simulink model "NavigationRocketPlant"  (R2025b)
settings: Solver=ode5  StartTime=0.0  StopTime=350  RelTol=1e-3
PostLoadFcn:
  | addpath('settings/')
  | addpath('settings/environment/')
  | 
  | run sensorSettings.m
InitFcn:
  | run(fullfile(fileparts(get_param(bdroot,'FileName')),'..','rocketPlantMain.m'))
values from neighbouring files (symbols this model uses):
  Rocket = block.DialogPrm(1).Data    [rocketPlantBlock.m]
  Weather = block.DialogPrm(3).Data    [rocketPlantBlock.m]
undefined symbols (not defined in the file or in its folder): ba0, bg0, DiscIntNeverNeededParam, dspblkCoreblockFVToolHelper, Environment, gcbh, GNSSConfig, GNSSInitialState, LLA0, MEKF, p0, P0, pressure0, q0, RocketInitialState, Sensor, stationaryTime, v0
libraries: simulink x2, dspmathops x1
(part 3 of 3)

== matlab function NavigationRocketPlant/Navigation/State Estimation/MEKF ==
  settings: updateMethod=DISCRETE  sampleTime=Sensor.Ts
  data: dt input; q_nb_out output; gyro_b input; acc_b input; baro_pressure_Pa input; mag_b input; h0_m input; gps_pos_n input; gps_fix_info input; mag_ref_n input; q_nb_in input; v_n_in input; p_n_in input; bg_in input; ba_in input; P_in input; use_acc_tilt input; mag_valid input; baro_valid input; gps_valid input; gps_frequency_Hz input; gps_timer_in input; v_n_out output; p_n_out output; bg_out output; ba_out output; P_out output; estimate_bias input; zeroUpdate input; gps_timer_out output; MEKF parameter; gps_diagnostic_out output; baro_calibration_out output double size=[2 1]; baro_calibration_in input double size=[2 1]; GNSSConfig parameter
function [q_nb_out, v_n_out, p_n_out, bg_out, ba_out, P_out, gps_timer_out, gps_diagnostic_out, baro_calibration_out] = MEKF_Navigation( ...
    dt, gyro_b, acc_b, baro_pressure_Pa, mag_b, h0_m, ...
    gps_pos_n, gps_fix_info, mag_ref_n, ...
    q_nb_in, v_n_in, p_n_in, bg_in, ba_in, P_in, ...
    use_acc_tilt, mag_valid, baro_valid, gps_valid, ...
    gps_frequency_Hz, gps_timer_in, ...
    estimate_bias, zeroUpdate, MEKF, baro_calibration_in, GNSSConfig)

    % -------------------------------------------------------------------------
    % Multiplicative Extended Kalman Filter for Navigation
    %
    % Sensors:
    %   gyro_b            : 3-axis gyroscope [rad/s]
    %   acc_b             : 3-axis accelerometer [m/s^2]
    %   mag_b             : 3-axis magnetometer [arbitrary unit or tesla]
    %   baro_pressure_Pa  : barometer pressure [Pa]
    %   gps_pos_n         : optional GPS position in local NED [m]
    %   gps_fix_info      : fresh/valid/acquisition time/age/NED sigma/status
    %   gps_frequency_Hz  : GPS update frequency [Hz]
    %   gps_timer_in      : last processed acquisition timestamp [s]
    %
    % Frame:
    %   n : local NED navigation frame
    %   b : body frame
    %
    % Quaternion:
    %   q_nb = [qx; qy; qz; qw], scalar-last
    %   q_nb maps body-frame vectors into navigation-frame vectors
    %
    % Nominal state:
    %   q_nb : attitude quaternion
    %   v_n  : velocity in NED [m/s]
    %   p_n  : position in NED [m]
    %   bg   : gyro bias [rad/s]
    %   ba   : accelerometer bias [m/s^2]
    %
    % Error state:
    %   dx = [dtheta; dv; dp; dbg; dba] in R^15
    %
    % Local NED convention:
    %   p_n(3) = D
    %   source-datum absolute altitude = h0_m - D
    %
    % -------------------------------------------------------------------------
    
    % -------------------------------------------------------------------------
    % Constants
    % -------------------------------------------------------------------------
    
    g0 = 9.80665;        % gravity magnitude [m/s^2]
    
    % -------------------------------------------------------------------------
    % Process diffusion tuning: Qd = G*Qc*G'*dt
    % -------------------------------------------------------------------------
    
    sigma_g = MEKF.sigma_g;
    sigma_a = MEKF.sigma_a;
    sigma_bg = MEKF.sigma_bg;
    sigma_ba = MEKF.sigma_ba;
    
    % -------------------------------------------------------------------------
    % Measurement-noise tuning
    % -------------------------------------------------------------------------
    
    sigma_acc_tilt = MEKF.sigma_acc_tilt;
    sigma_mag = MEKF.sigma_mag;
    sigma_baro_p = MEKF.sigma_baro_p;
    
    % Accelerometer update gate.
    % Accelerometer is used as gravity direction only when norm is close to g.
    acc_gate = MEKF.acc_gate;
    
    % -------------------------------------------------------------------------
    % Input protection
    % -------------------------------------------------------------------------
    
    if dt <= 0.0
        dt = 1.0e-3;
    end

    % -------------------------------------------------------------------------
    % GNSS delivery and duplicate/stale protection
    % -------------------------------------------------------------------------
    % A held receiver position is not a fresh measurement. Use the delivered
    % packet flags and timestamp, rather than a second independent 10 Hz timer.
    % Initialize the last processed timestamp to -1 so epoch zero is accepted.
    gps_timer = gps_timer_in;
    gps_update = 0;
    gps_age = gps_fix_info(4);
    gps_diagnostic = [0.0; 0.0; 0.0; gps_age];
    if gps_valid && gps_frequency_Hz > 0.0 && ...
            gps_fix_info(1) > 0.5 && gps_fix_info(2) > 0.5 && ...
            all(isfinite(gps_fix_info)) && gps_age >= 0.0 && ...
            gps_age <= GNSSConfig.MaxAge && ...
            gps_fix_info(3) > gps_timer_in + 1.0e-9 && ...
            all(gps_fix_info(5:7) >= 0.0)
        gps_update = 1;
        gps_timer = gps_fix_info(3);
        gps_diagnostic(1) = 1.0;
    end
    
    q_nb = quatNormalize(q_nb_in);
    v_n  = v_n_in;
    p_n  = p_n_in;
    bg   = bg_in;
    ba   = ba_in;
    

    P = 0.5 * (P_in + P_in');
    % Startup pressure zeroing at the known local origin.
    % Explicit Unit Delay state [offset_Pa; sample_count], initially [0;0].
    % Reset each simulation; freeze at launch. No sensor truth is used.
    baro_offset_Pa = baro_calibration_in(1);
    baro_samples = baro_calibration_in(2);
    if MEKF.baro_zero_enabled && zeroUpdate && baro_valid && isfinite(baro_pressure_Pa)
        [p_origin, ~] = ISA_model(0.0, h0_m);
        baro_samples = baro_samples + 1.0;
        baro_offset_Pa = baro_offset_Pa + ...
            (baro_pressure_Pa - p_origin - baro_offset_Pa) / baro_samples;
    end
    baro_pressure_calibrated = baro_pressure_Pa;
    if MEKF.baro_zero_enabled
        baro_pressure_calibrated = baro_pressure_Pa - baro_offset_Pa;
    end
    baro_calibration_out = [baro_offset_Pa; baro_samples];

    
    % -------------------------------------------------------------------------
    % Prediction step
    % -------------------------------------------------------------------------
    
    omega_b = gyro_b - bg;
    f_b     = acc_b  - ba;
    
    % Quaternion propagation.
    dq = deltaQuat(omega_b * dt);
    q_nb = quatNormalize(quatMultiply(q_nb, dq));
    
    % Rotation matrix from body frame to navigation frame.
    C_nb = quatToDcm(q_nb);
    
    % Strapdown translational propagation.
    % In NED, gravity is positive in the Down direction.
    g_n = [0.0; 0.0; g0];
    
    a_n = C_nb * f_b + g_n;
    
    p_n = p_n + v_n * dt + 0.5 * a_n * dt * dt;
    v_n = v_n + a_n * dt;
    
    % -------------------------------------------------------------------------
    % Covariance prediction
    % -------------------------------------------------------------------------
    
    F = zeros(15,15);
    
    % Attitude error dynamics:
    % dtheta_dot = -skew(omega_b) dtheta - dbg
    F(1:3,1:3)   = -skew3(omega_b);
    F(1:3,10:12) = -eye(3);
    
    % Velocity error dynamics:
    % dv_dot = -C_nb skew(f_b) dtheta - C_nb dba
    F(4:6,1:3)   = -C_nb * skew3(f_b);
    F(4:6,13:15) = -C_nb;
    
    % Position error dynamics:
    % dp_dot = dv
    F(7:9,4:6) = eye(3);
    
    % Bias dynamics:
    %   bg_dot = n_bg
    %   ba_dot = n_ba
    
    Phi = eye(15) + F * dt;
    
    G = zeros(15,12);
    
    G(1:3,1:3)     = -eye(3);   % gyro noise
    G(4:6,4:6)     = -C_nb;     % accelerometer noise
    G(10:12,7:9)   = eye(3);    % gyro bias random walk
    G(13:15,10:12) = eye(3);    % accelerometer bias random walk
    
    Qc = zeros(12,12);
    
    Qc(1:3,1:3)     = sigma_g^2  * eye(3);
    Qc(4:6,4:6)     = sigma_a^2  * eye(3);
    Qc(7:9,7:9)     = sigma_bg^2 * eye(3);
    Qc(10:12,10:12) = sigma_ba^2 * eye(3);
    
    Qd = G * Qc * G' * dt;
    
    P = Phi * P * Phi' + Qd;
    P = 0.5 * (P + P');

    
    if zeroUpdate
    
        [q_nb, v_n, p_n, bg, ba, P] = ZeroUpdateKalmanFilter( ...
            gyro_b, acc_b, q_nb, v_n, p_n, bg, ba, P, g0, estimate_bias, MEKF);
    
        C_nb = quatToDcm(q_nb);
    
    end

    % -------------------------------------------------------------------------
    % Accelerometer attitude update
    % -------------------------------------------------------------------------
    % The accelerometer update is used only when the acceleration norm is close
    % to gravity. Otherwise, the accelerometer contains significant translational
    % acceleration and should not be treated as a gravity vector.
    
    % Use the corrected bias; do not reuse the pre-zero-update value.
    f_b = acc_b - ba;
    acc_norm = norm3(f_b);
    
    if use_acc_tilt && ~zeroUpdate && acc_norm > 1.0e-6
    
        if abs(acc_norm - g0) < acc_gate * g0
    
            y_acc = f_b / acc_norm;
    
            C_bn = C_nb';
    
            g_unit_n = [0.0; 0.0; 1.0];
    
            % At rest, accelerometer measures approximately -gravity direction.
            yhat_acc = -C_bn * g_unit_n;
    
            H_acc = zeros(3,15);
            H_acc(:,1:3) = skew3(yhat_acc);
    
            [q_nb, v_n, p_n, bg, ba, P] = updateVector3( ...
                y_acc, yhat_acc, H_acc, sigma_acc_tilt^2, ...
                q_nb, v_n, p_n, bg, ba, P, estimate_bias);
    
            C_nb = quatToDcm(q_nb);
        end
    end
    
    % -------------------------------------------------------------------------
    % Magnetometer attitude update
    % -------------------------------------------------------------------------
    % Magnetometer measurement model:
    %
    %   z_m    = normalized measured magnetic field in body frame
    %   zhat_m = C_bn * m_ref_n
    %
    % where m_ref_n is the reference magnetic field in the navigation frame.
    
    mag_norm = norm3(mag_b);
    mag_ref_norm = norm3(mag_ref_n);
    
    if mag_valid && mag_norm > 1.0e-6 && mag_ref_norm > 1.0e-6
    
        y_mag = mag_b / mag_norm;
        m_ref_n = mag_ref_n / mag_ref_norm;
    
        C_bn = C_nb';
    
        yhat_mag = C_bn * m_ref_n;
    
        H_mag = zeros(3,15);
        H_mag(:,1:3) = skew3(yhat_mag);
    
        [q_nb, v_n, p_n, bg, ba, P] = updateVector3( ...
            y_mag, yhat_mag, H_mag, sigma_mag^2, ...
            q_nb, v_n, p_n, bg, ba, P, estimate_bias);
    
        C_nb = quatToDcm(q_nb);
    end
    
    % -------------------------------------------------------------------------
    % Barometer EKF update
    % -------------------------------------------------------------------------
    % The barometer is treated as a pressure sensor.
    %
    % Nonlinear measurement model:
    %
    %   z_b    = p_baro
    %   zhat_b = p_ISA(D)
    %
    % where:
    %
    %   D = p_n(3)
    %   h = h0_m - D
    %
    % The measurement Jacobian is:
    %
    %   H_b = dp_ISA/dD
    %
    % Since the error state contains dp at indices 7:9, the Down-position
    % derivative enters column 9.
    
    if baro_valid && isfinite(baro_pressure_calibrated)
    
        [p_hat, dp_dD] = ISA_model(p_n(3), h0_m);
    
        H_baro = zeros(1,15);
        H_baro(1,9) = dp_dD;
    
        [q_nb, v_n, p_n, bg, ba, P] = updateScalar( ...
            baro_pressure_calibrated, p_hat, H_baro, sigma_baro_p^2, ...
            q_nb, v_n, p_n, bg, ba, P, estimate_bias);
    
        C_nb = quatToDcm(q_nb);
    end
    
    % -------------------------------------------------------------------------
    % Optional GPS update
    % -------------------------------------------------------------------------

    if gps_update && all(isfinite(gps_pos_n))

        z_gps = gps_pos_n;
        % Short-latency kinematic observation at the acquisition time.
        % Uses Navigation's own state, never GNSS velocity or trajectory truth.
        % This bounded approximation is not a fixed-lag replay filter.
        acceleration_now = C_nb * (acc_b - ba) + [0.0;0.0;g0];
        zhat_gps = p_n - v_n * gps_age + ...
            0.5 * acceleration_now * gps_age^2;
        H_gps = zeros(3,15);
        H_gps(:,1:3) = -0.5 * gps_age^2 * C_nb * skew3(acc_b - ba);
        H_gps(:,4:6) = -gps_age * eye(3);
        H_gps(:,7:9) = eye(3);
        H_gps(:,13:15) = -0.5 * gps_age^2 * C_nb;
        latency_sigma = 0.5 * GNSSConfig.Navigation.LatencyAccelerationSigma * gps_age^2;
        % Per-fix metric uncertainty includes white, slow and multipath terms.
        % Keep a finite numerical floor for deliberately noiseless test cases.
        R_gps = diag(max(gps_fix_info(5:7).^2 + latency_sigma^2,1.0e-8));
        residual_gps = z_gps - zhat_gps;
        innovation_covariance = H_gps * P * H_gps' + R_gps;
        gps_nis = residual_gps' * (innovation_covariance \ residual_gps);
        gps_diagnostic(3) = gps_nis;
        % Reject the entire GNSS correction for a large outlier. This differs
        % from the existing bias-learning gate, which only protects ba.
        if isfinite(gps_nis) && gps_nis <= GNSSConfig.Navigation.NISLimit
        gps_diagnostic(2) = 1.0;

        % Position residuals can observe accelerometer bias through the
        % propagated p-v-ba covariance. Do not use GPS velocity or truth.
        learn_acc_bias = estimate_bias || (MEKF.acc_bias_flight_enabled && ...
            ~zeroUpdate && all(isfinite(f_b)) && ...
            norm3(f_b) <= MEKF.acc_bias_force_max);
        if estimate_bias
            bias_step_limit = inf;
            bias_nis_limit = inf;
        else
            bias_step_limit = MEKF.acc_bias_max_rate * ...
                max(dt, 1.0 / gps_frequency_Hz);
            bias_nis_limit = MEKF.acc_bias_nis_max;
        end

        [q_nb, v_n, p_n, bg, ba, P] = updateVector3( ...
            z_gps, zhat_gps, H_gps, R_gps, ...
            q_nb, v_n, p_n, bg, ba, P, estimate_bias, ...
            learn_acc_bias, bias_step_limit, bias_nis_limit);
        if learn_acc_bias && ~estimate_bias
            % Uncalibrated gain/alignment errors are not random-walk bias.
            % Retain an uncertainty allowance instead of becoming overconfident.
            % Adding only a nonnegative diagonal preserves covariance PSD.
            for axis = 1:3
                index = 12 + axis;
                P(index,index) = max(P(index,index), ...
                    MEKF.acc_bias_variance_floor);
            end
        end
        C_nb = quatToDcm(q_nb);
        end
    end

    % Outputs
    % -------------------------------------------------------------------------
    
    q_nb_out = quatNormalize(q_nb);
    v_n_out  = v_n;
    p_n_out  = p_n;
    bg_out   = bg;
    ba_out   = ba;
    P_out    = 0.5 * (P + P');
    gps_timer_out = gps_timer;
    gps_diagnostic_out = gps_diagnostic; % [fresh valid request; accepted; NIS; age]
    
end


%% Zero Update Kalman Filter
function [q, v, p, bg, ba, P] = ZeroUpdateKalmanFilter(gyro_b, acc_b, q, v, p, bg, ba, P, g0, estimate_bias, MEKF)


    % -------------------------------------------------------------------------
    % Stationary zero-update Kalman correction for MEKF
    %
    % This block assumes:
    %   - the sensor is not translating
    %   - the sensor is not rotating
    %   - velocity should be zero
    %   - accelerometer measures only gravity plus bias
    %   - gyroscope measures only bias
    %
    % State error:
    %   dx = [dtheta; dv; dp; dbg; dba]
    % -------------------------------------------------------------------------
    
    % Tuning values.
    % Start conservative, then reduce after checking residuals.
    sigma_zupt_v = MEKF.sigma_zupt_v;
    sigma_zaru_g = MEKF.sigma_zaru_g;
    sigma_acc_b = MEKF.sigma_acc_b;
    sigma_zp_p = MEKF.sigma_zp_p;
    
    % -------------------------------------------------------------------------
    % 1) Zero-velocity update, ZUPT
    % -------------------------------------------------------------------------
    % Measurement:
    %   z_v = 0
    %   zhat_v = v
    %
    % Jacobian:
    %   H_v = [0 I 0 0 0]
    
    z_zupt = zeros(3,1);
    zhat_zupt = v;
    
    H_zupt = zeros(3,15);
    H_zupt(:,4:6) = eye(3);
    
    [q, v, p, bg, ba, P] = updateVector3( ...
        z_zupt, zhat_zupt, H_zupt, sigma_zupt_v^2, ...
        q, v, p, bg, ba, P, estimate_bias);
    
    % -------------------------------------------------------------------------
    % 2) Zero-angular-rate update, ZARU
    % -------------------------------------------------------------------------
    % Stationary gyroscope model:
    %   gyro_b = bg + noise
    %
    % Measurement:
    %   z_g = gyro_b
    %   zhat_g = bg
    %
    % Jacobian:
    %   H_g = [0 0 0 I 0]
    
    z_zaru = gyro_b;
    zhat_zaru = bg;
    
    H_zaru = zeros(3,15);
    H_zaru(:,10:12) = eye(3);
    
    [q, v, p, bg, ba, P] = updateVector3( ...
        z_zaru, zhat_zaru, H_zaru, sigma_zaru_g^2, ...
        q, v, p, bg, ba, P, estimate_bias);
    
    % -------------------------------------------------------------------------
    % 3) Stationary accelerometer-bias update
    % -------------------------------------------------------------------------
    % Stationary accelerometer model:
    %   acc_b = -C_bn*g_n + ba + noise
    %
    % This is the update that directly helps accelerometer-bias convergence.
    %
    % Measurement:
    %   z_a = acc_b
    %   zhat_a = -C_bn*g_n + ba
    %
    % Jacobian:
    %   H_a = [d(acc)/dtheta, 0, 0, 0, I]
    
    C_nb = quatToDcm(q);
    C_bn = C_nb';
    
    g_n = [0.0; 0.0; g0];
    
    f_grav_b = -C_bn * g_n;
    
    z_acc = acc_b;
    zhat_acc = f_grav_b + ba;
    
    H_acc = zeros(3,15);
    
    % Attitude sensitivity.
    % This sign is consistent with the attitude-error convention used in the
    % previous accelerometer and magnetometer updates.
    H_acc(:,1:3) = skew3(f_grav_b);
    
    % Direct accelerometer-bias sensitivity.
    H_acc(:,13:15) = eye(3);
    
    [q, v, p, bg, ba, P] = updateVector3( ...
        z_acc, zhat_acc, H_acc, sigma_acc_b^2, ...
        q, v, p, bg, ba, P, estimate_bias);
    
    % -------------------------------------------------------------------------
    % 4) Zero-Position update
    % -------------------------------------------------------------------------
    % Use this only if the sensor is fixed at the local origin during the stationary phase.

    z_zp = [0; 0; 0];
    zhat_zp = p;

    H_zp = zeros(3,15);
    H_zp(:,7:9) = eye(3);

    [q, v, p, bg, ba, P] = updateVector3( ...
        z_zp, zhat_zp, H_zp, sigma_zp_p^2, ...
        q, v, p, bg, ba, P, estimate_bias);

end

== matlab function NavigationRocketPlant/Navigation/NED to LLA ==
  data: p_N input; LLA output; LLA0 input
function LLA = NED2LLA(p_N, LLA0)

    % p_N  = [north; east; down] in meters
    % LLA0 = [lat0; lon0; h0]
    % lat0, lon0 in rad
    % h0 in m
    %
    % LLA output = [lat; lon; h]
    % lat, lon in rad
    % h in m
    
    % WGS-84 constants
    a = 6378137.0;
    e2 = 6.69437999014e-3;
    
    lat0 = LLA0(1);
    lon0 = LLA0(2);
    h0   = LLA0(3);
    
    north = p_N(1);
    east  = p_N(2);
    down = p_N(3);
    
    sinLat = sin(lat0);
    
    RN = a / sqrt(1 - e2*sinLat^2);
    RM = a*(1 - e2) / (1 - e2*sinLat^2)^(3/2);
    
    lat = lat0 + north/(RM + h0);
    lon = lon0 + east/((RN + h0)*cos(lat0));
    h   = h0 - down;
    
    LLA = [lat; lon; h];

end

== matlab function NavigationRocketPlant/Enviroment/System/MATLAB Function ==
  data: h input; p output
function p = ISA_altitude_to_pressure(h)

    % ISA altitude-to-pressure conversion for the troposphere.
    %
    % Input:
    %   h : altitude above sea level [m]
    %
    % Output:
    %   p : static pressure [Pa]
    %
    % Assumptions:
    %   - ISA troposphere model
    %   - sea-level pressure p0 = 101325 Pa
    %   - valid approximately for h < 11 km
    
    T0 = 288.15;       % sea-level standard temperature [K]
    L  = 0.0065;       % temperature lapse rate [K/m]
    R  = 287.05;       % specific gas constant for air [J/(kg K)]
    g0 = 9.80665;      % gravitational acceleration [m/s^2]
    p0 = 101325.0;     % sea-level standard pressure [Pa]
    
    exponent = g0 / (R * L);
    
    p = p0 * (1.0 - (L * h) / T0)^exponent;

end
